simulink model "state_space_model"  (R2018b)
settings: Solver=VariableStepAuto  StartTime=0.0  StopTime=1  RelTol=1e-3
values from neighbouring files (symbols this model uses):
  A = [ ... (first row only)    [lecture_ODE_to_state_space.m]
  B = [ ... (first row only)    [lecture_ODE_to_state_space.m]
  C = [ ... (first row only)    [lecture_ODE_to_state_space.m]
  D = [ ... (first row only)    [lecture_ODE_to_state_space.m]
  x0 = [ ... (first row only)    [lecture_ODE_to_state_space.m]
settings Model: Creator=Christopher  LastModifiedBy=Christopher

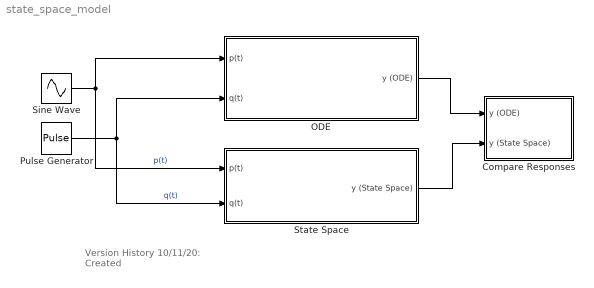
== system state_space_model ==
  note: Version History
      | 10/11/20: Created
  Compare Responses : Subsystem
  ODE : Subsystem
  Pulse Generator : DiscretePulseGenerator  PulseType=Time based  Period=0.1  PulseWidth=25
  Sine Wave : Sin  SampleTime=0
  State Space : Subsystem
  wires:
  Sine Wave/1 -> ODE/1(p(t)), State Space/1(p(t))  "p(t)"
  Pulse Generator/1 -> ODE/2(q(t)), State Space/2(q(t))  "q(t)"
  ODE/1(y (ODE)) -> Compare Responses/1(y (ODE))
  State Space/1(y (State Space)) -> Compare Responses/2(y (State Space))

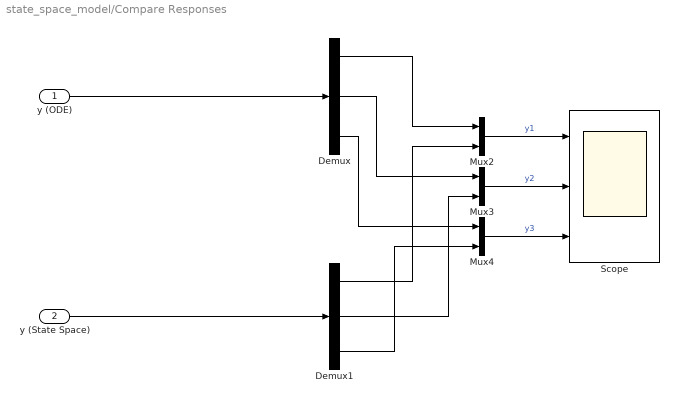
== system state_space_model/Compare Responses ==
  y (ODE) : Inport
  y (State Space) : Inport  Port=2
  Demux : Demux  Outputs=3
  Demux1 : Demux  Outputs=3
  Mux2 : Mux  Inputs=2
  Mux3 : Mux  Inputs=2
  Mux4 : Mux  Inputs=2
  Scope : Scope  NumInputPorts=3
  wires:
  Mux4/1 -> Scope/3  "y3"
  Demux1/3 -> Mux4/2
  Mux2/1 -> Scope/1  "y1"
  Demux1/1 -> Mux2/2
  Demux/2 -> Mux3/1
  Demux1/2 -> Mux3/2
  Demux/3 -> Mux4/1
  y (State Space)/1 -> Demux1/1
  Demux/1 -> Mux2/1
  Mux3/1 -> Scope/2  "y2"
  y (ODE)/1 -> Demux/1

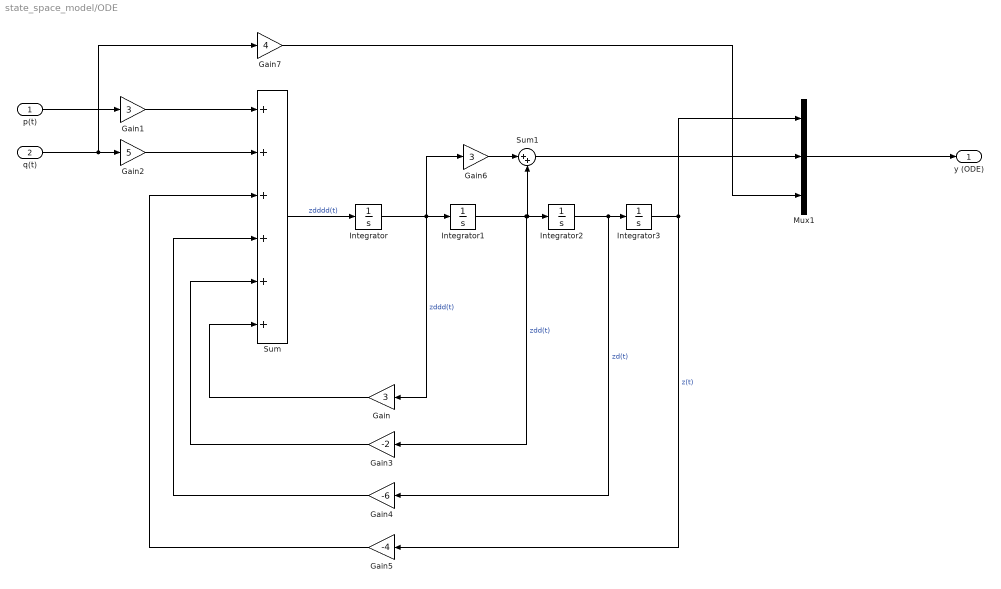
== system state_space_model/ODE ==
  p(t) : Inport
  q(t) : Inport  Port=2
  Gain : Gain  Gain=3
  Gain1 : Gain  Gain=3
  Gain2 : Gain  Gain=5
  Gain3 : Gain  Gain=-2
  Gain4 : Gain  Gain=-6
  Gain5 : Gain  Gain=-4
  Gain6 : Gain  Gain=3
  Gain7 : Gain  Gain=4
  Integrator : Integrator  InitialCondition=x0(4)
  Integrator1 : Integrator  InitialCondition=x0(3)
  Integrator2 : Integrator  InitialCondition=x0(2)
  Integrator3 : Integrator  InitialCondition=x0(1)
  Mux1 : Mux  Inputs=3
  Sum : Sum  Inputs=++++++
  Sum1 : Sum  Inputs=|++
  y (ODE) : Outport
  wires:
  Gain1/1 -> Sum/1
  Integrator3/1 -> Mux1/1, Gain5/1  "z(t)"
  Gain2/1 -> Sum/2
  Integrator2/1 -> Gain4/1, Integrator3/1  "zd(t)"
  Sum/1 -> Integrator/1  "zdddd(t)"
  Integrator/1 -> Gain6/1, Gain/1, Integrator1/1  "zddd(t)"
  Gain4/1 -> Sum/4
  Mux1/1 -> y (ODE)/1
  Integrator1/1 -> Sum1/2, Integrator2/1, Gain3/1  "zdd(t)"
  q(t)/1 -> Gain7/1, Gain2/1
  Gain6/1 -> Sum1/1
  Gain3/1 -> Sum/5
  Gain/1 -> Sum/6
  p(t)/1 -> Gain1/1
  Gain7/1 -> Mux1/3
  Sum1/1 -> Mux1/2
  Gain5/1 -> Sum/3

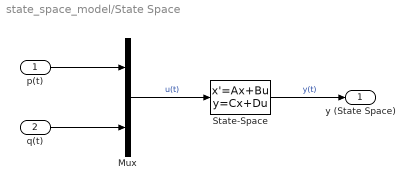
== system state_space_model/State Space ==
  p(t) : Inport
  q(t) : Inport  Port=2
  Mux : Mux  Inputs=2
  State-Space : StateSpace  A=A  B=B  C=C  D=D  InitialCondition=x0
  y (State Space) : Outport
  wires:
  p(t)/1 -> Mux/1
  q(t)/1 -> Mux/2
  Mux/1 -> State-Space/1  "u(t)"
  State-Space/1 -> y (State Space)/1  "y(t)"
